simulink model "controlTest3"  (R2017b)
settings: Solver=VariableStepAuto  StartTime=0.0  StopTime=1000  RelTol=1e-3
libraries: cstblocks x2
settings Model: Creator=youxu  LastModifiedBy=youxu

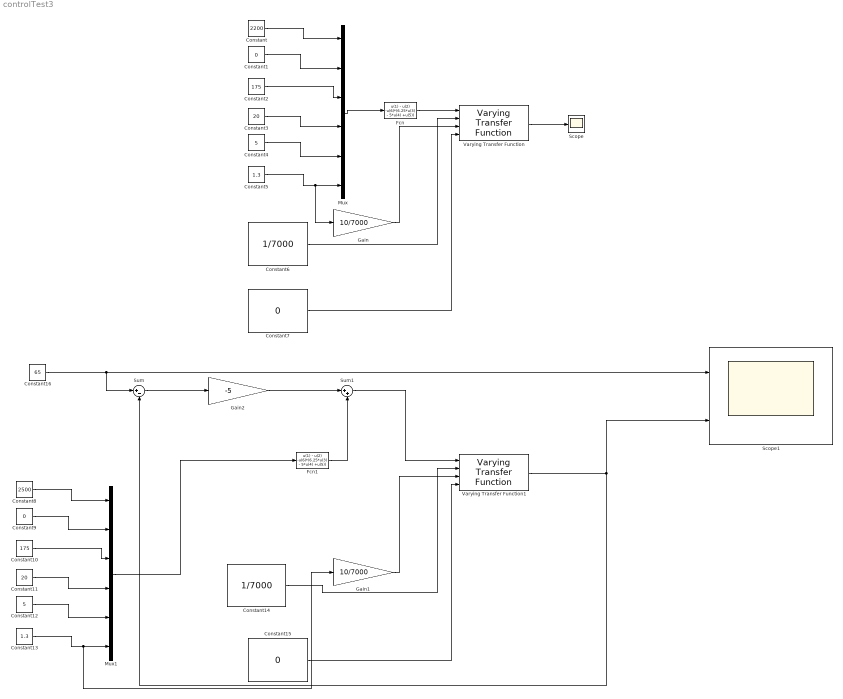
== system controlTest3 ==
  Constant : Constant  Value=2200
  Constant{1,7,9,15} (4 alike) : Constant  Value=0
  Constant10 : Constant  Value=175
  Constant11 : Constant  Value=20
  Constant12 : Constant  Value=5
  Constant13 : Constant  Value=1.3
  Constant14 : Constant  Value=1/7000
  Constant16 : Constant  Value=65
  Constant2 : Constant  Value=175
  Constant3 : Constant  Value=20
  Constant4 : Constant  Value=5
  Constant5 : Constant  Value=1.3
  Constant6 : Constant  Value=1/7000
  Constant8 : Constant  Value=2500
  Fcn : Fcn  Expr=u(1) - u(2) -u(6)*(6.25*u(3) - 5*u(4) +u(5))
  Fcn1 : Fcn  Expr=u(1) - u(2) -u(6)*(6.25*u(3) - 5*u(4) +u(5))
  Gain : Gain  Gain=10/7000
  Gain1 : Gain  Gain=10/7000
  Gain2 : Gain  Gain=-5
  Mux : Mux  Inputs=6
  Mux1 : Mux  Inputs=6
  Scope : Scope
  Scope1 : Scope  NumInputPorts=2
  Sum : Sum  Inputs=|+-
  Sum1 : Sum  Inputs=|++
  Varying Transfer Function : cstblocks/Linear Parameter Varying/Varying Transfer Function  N=1
      link override Integrator1: InitialCondition=70
      settings: SourceProductName=Control System Toolbox
  Varying Transfer Function1 : cstblocks/Linear Parameter Varying/Varying Transfer Function  N=1
      link override Integrator1: InitialCondition=70
      settings: SourceProductName=Control System Toolbox
  wires:
  Constant/1 -> Mux/1
  Constant1/1 -> Mux/2
  Constant2/1 -> Mux/3
  Constant3/1 -> Mux/4
  Constant4/1 -> Mux/5
  Constant5/1 -> Gain/1, Mux/6
  Mux/1 -> Fcn/1
  Fcn/1 -> Varying Transfer Function/1
  Varying Transfer Function/1 -> Scope/1
  Constant6/1 -> Varying Transfer Function/2
  Constant7/1 -> Varying Transfer Function/4
  Gain/1 -> Varying Transfer Function/3
  Gain1/1 -> Varying Transfer Function1/3
  Constant15/1 -> Varying Transfer Function1/4
  Constant14/1 -> Varying Transfer Function1/2
  Varying Transfer Function1/1 -> Sum/2, Scope1/2
  Mux1/1 -> Fcn1/1
  Constant13/1 -> Mux1/6, Gain1/1
  Constant12/1 -> Mux1/5
  Constant11/1 -> Mux1/4
  Constant10/1 -> Mux1/3
  Constant9/1 -> Mux1/2
  Constant8/1 -> Mux1/1
  Constant16/1 -> Sum/1, Scope1/1
  Sum/1 -> Gain2/1
  Gain2/1 -> Sum1/1
  Fcn1/1 -> Sum1/2
  Sum1/1 -> Varying Transfer Function1/1
